simulink model "subs_MM"  (R2018b)
settings: Solver=VariableStepAuto  StartTime=0.0  StopTime=inf  FixedStep=0.01  RelTol=1e-3
InitFcn:
  | clear
undefined symbols (not defined in the file or in its folder): Angular, Linear
libraries: robotlib x3
settings Model: Creator=francesco  LastModifiedBy=francesco

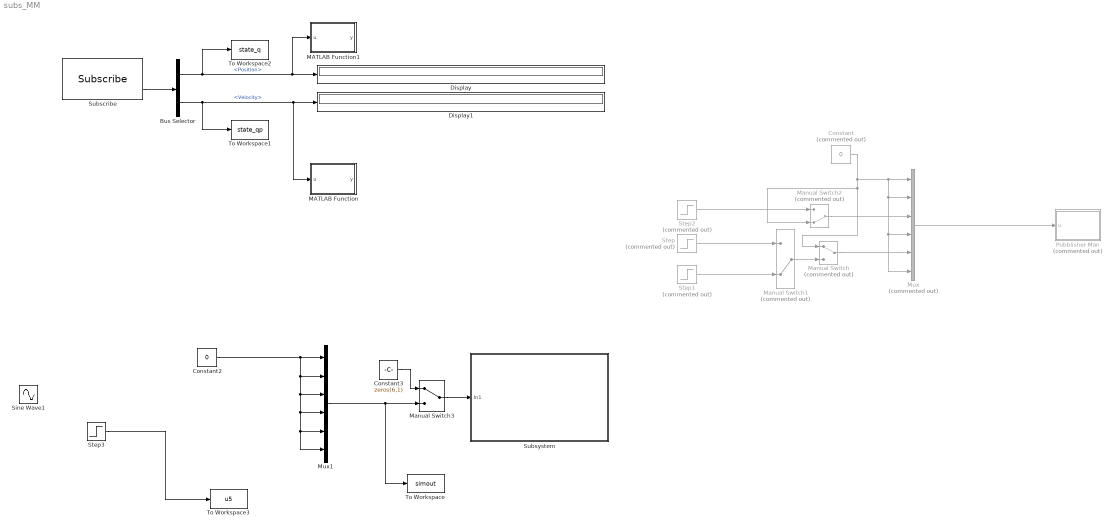
== system subs_MM ==
  Bus Selector : BusSelector  OutputSignals=Position,Velocity
  Constant : Constant  Commented=on  Value=0
  Constant2 : Constant  Value=0
  Constant3 : Constant  Value=zeros(6,1)
  Display : Display
  Display1 : Display
  MATLAB Function : MATLAB Function  TreatAsAtomicUnit=on
  MATLAB Function1 : MATLAB Function  TreatAsAtomicUnit=on
  Manual Switch : ManualSwitch  Commented=on
  Manual Switch1 : ManualSwitch  Commented=on  CurrentSetting=0
  Manual Switch2 : ManualSwitch  Commented=on  CurrentSetting=0
  Manual Switch3 : ManualSwitch
  Mux : Mux  Commented=on  Inputs=6
  Mux1 : Mux  Inputs=6
  Pubblisher Man : MATLAB Function  Commented=on  TreatAsAtomicUnit=on
  Sine Wave1 : Sin  Amplitude=0.3  Frequency=0.05  SampleTime=0
  Step : Step  Commented=on  Time=0  After=0.3  SampleTime=0
  Step1 : Step  Commented=on  Time=0  After=-0.3  SampleTime=0
  Step2 : Step  Commented=on  Time=0  After=--0.1  SampleTime=0
  Step3 : Step  Time=0  After=0.2  SampleTime=0
  Subscribe : robotlib/Subscribe  topicSource=Select from ROS network  topic=/joint_states  messageType=sensor_msgs/JointState  sampleTime=-1  messageQueueLength=1
      settings: SourceProductBaseCode=RO
  Subsystem : Subsystem
  To Workspace : ToWorkspace  VariableName=simout  SampleTime=-1
  To Workspace1 : ToWorkspace  VariableName=state_qp  SampleTime=-1
  To Workspace2 : ToWorkspace  VariableName=state_q  SampleTime=-1
  To Workspace3 : ToWorkspace  VariableName=u5  SampleTime=-1
  wires:
  Constant/1 -> Manual Switch/1, Manual Switch2/2, Mux/2, Mux/6, Mux/4, Mux/1
  Subscribe/2 -> Bus Selector/1
  Bus Selector/2 -> MATLAB Function/1(u), Display1/1, To Workspace1/1  "<Velocity>"
  Bus Selector/1 -> To Workspace2/1, MATLAB Function1/1(u), Display/1  "<Position>"
  Manual Switch/1 -> Mux/5
  Step1/1 -> Manual Switch1/2
  Step/1 -> Manual Switch1/1
  Manual Switch1/1 -> Manual Switch/2
  Manual Switch2/1 -> Mux/3
  Step2/1 -> Manual Switch2/1
  Mux/1 -> Pubblisher Man/1(u)
  Manual Switch3/1 -> Subsystem/1(In1)
  Mux1/1 -> To Workspace/1, Manual Switch3/2
  Constant3/1 -> Manual Switch3/1
  Constant2/1 -> Mux1/1, Mux1/5, Mux1/6, Mux1/4, Mux1/3, Mux1/2
  Step3/1 -> To Workspace3/1

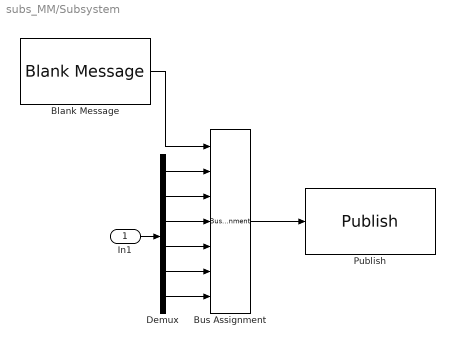
== system subs_MM/Subsystem ==
  In1 : Inport
  Blank Message : robotlib/Blank Message  messageClass=Message  entityType=geometry_msgs/Twist  messageType=geometry_msgs/Twist  SampleTime=inf
      settings: SourceProductBaseCode=RO
  Bus Assignment : BusAssignment  AssignedSignals=Linear.X,Linear.Y,Linear.Z,Angular.X,Angular.Y,Angular.Z
  Demux : Demux  Outputs=6
  Publish : robotlib/Publish  topicSource=Select from ROS network  topic=/control_c  messageType=geometry_msgs/Twist  messageQueueLength=1
      settings: SourceProductBaseCode=RO
  wires:
  Demux/2 -> Bus Assignment/3
  Demux/3 -> Bus Assignment/4
  Demux/5 -> Bus Assignment/6
  Blank Message/1 -> Bus Assignment/1
  Demux/1 -> Bus Assignment/2
  Demux/6 -> Bus Assignment/7
  Bus Assignment/1 -> Publish/1
  In1/1 -> Demux/1
  Demux/4 -> Bus Assignment/5

== matlab function subs_MM/MATLAB Function ==
  data: u input; y output
function y = fcn(u)

y = u(1:6);

== matlab function subs_MM/Pubblisher Man ==
  settings: sampleTime=1/23000
  data: u input
function fcn(u)
coder.extrinsic('publisherMM')

publisherMM(u);

end

== matlab function subs_MM/MATLAB Function1 ==
  data: u input; y output
function y = fcn(u)

y = u(1:6);
